simulink library "Lib_JMplatform_deVCU_Com"  (R2019b)
settings: Solver=ode45  StartTime=0.0  StopTime=10.0  RelTol=1e-3  EnableMultiTasking=on
settings Model: Creator=kmansour  LastModifiedBy=User
settings DataIOCC: LimitDataPoints=on  SaveFormat=Array  ReturnWorkspaceOutputs=off
settings OptimizationCC: LifeSpan=inf
settings DebuggingCC: AllowSymbolicDim=off  SFUnexpectedBacktrackingDiag=warning  SFNoUnconditionalDefaultTransitionDiag=warning  SFExecutionAtInitializationDiag=none  ArithmeticOperatorsInVariantConditions=warning
settings HardwareCC: ProdBitPerPointer=32  ProdBitPerSizeT=32  ProdBitPerPtrDiffT=32  ProdLargestAtomicFloat=None  ProdIntDivRoundTo=Undefined  ProdEndianess=Unspecified  ProdWordSize=32  ProdHWDeviceType=32-bit Generic
settings ModelReferenceCC: PropagateSignalLabelsOutOfModel=off
settings SFSimCC: SimUseLocalCustomCode=off  CustomCodeUndefinedFunction=UseInterfaceOnly
settings RTWCC: RTWUseLocalCustomCode=off
settings CodeAppCC: StateflowObjectComments=on
settings GRTTargetCC: TargetLangStandard=C89/C90 (ANSI)  GeneratePreprocessorConditionals=Disable all
settings ConfigComp: CovMetricSettings=dw  CovHtmlReporting=on  CovSaveCumulativeToWorkspaceVar=on  CovSaveSingleToWorkspaceVar=on  CovExternalEMLEnable=off

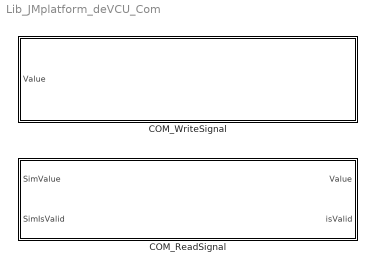
== system Lib_JMplatform_deVCU_Com ==
  COM_ReadSignal : Subsystem  TreatAsAtomicUnit=on  mask{PARAM_ID=APP_RX_CAN1TESTRX1}
      mask prompts: PARAM_ID "Choose Signal"
      mask TypeOptions PARAM_ID: APP_RX_CAN1TESTRX1 | APP_RX_CAN2TESTRX1 | APP_RX_CAN3TESTRX1
      mask Display:
      | image(imread('devcu_final.png'),'top-left');
      | color('black');
      | port_label('input', 1, 'SimValue');
      | port_label('input', 2, 'SimIsValid');
      | port_label('output', 1, 'Value');
      | port_label('output', 2, 'isValid');
      | 
      | strCell =get_param(gcb, 'MaskValues');
      | strCell = strtrim(strCell);
      | str = strCell{1};
      | str = strrep(str, '_', '\_');
      | disp(str, 'texmode', 'on');
  COM_WriteSignal : Subsystem  TreatAsAtomicUnit=on  mask{PARAM_ID=APP_TX_CAN1TESTTX1}
      mask prompts: PARAM_ID "Choose Signal"
      mask TypeOptions PARAM_ID: APP_TX_CAN1TESTTX1 | APP_TX_CAN2TESTTX2 | APP_TX_CAN3TEXTTX1
      mask Display:
      | image(imread('devcu_final.png'),'top-right');
      | color('black');
      | port_label('input', 1, 'Value');
      | 
      | strCell =get_param(gcb, 'MaskValues');
      | strCell = strtrim(strCell);
      | str = strCell{1};
      | str = strrep(str, '_', '\_');
      | disp(str, 'texmode', 'on');

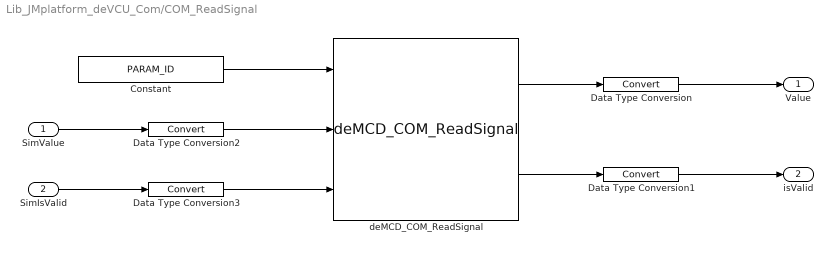
== system Lib_JMplatform_deVCU_Com/COM_ReadSignal ==
  SimValue : Inport
  SimIsValid : Inport  Port=2
  Constant : Constant  Value=PARAM_ID
  Data Type Conversion{,1..3} (4 alike) : DataTypeConversion
  deMCD_COM_ReadSignal : S-Function  FunctionName=deMCD_COM_ReadSignal  SFunctionDeploymentMode=off  EnableBusSupport=off
      mask Display:
      | image(imread('logo_deMCD_white_background.png'),'center');
      | color('black');
      | port_label('input', 1, 'ID');
      | port_label('input', 2, 'SimValue');
      | port_label('input', 3, 'SimIsValid');
      | port_label('output', 1, 'Value');
      | port_label('output', 2, 'isValid');
  Value : Outport
  isValid : Outport  Port=2
  wires:
  Constant/1 -> deMCD_COM_ReadSignal/1
  deMCD_COM_ReadSignal/1 -> Data Type Conversion/1
  deMCD_COM_ReadSignal/2 -> Data Type Conversion1/1
  Data Type Conversion/1 -> Value/1
  Data Type Conversion1/1 -> isValid/1
  SimValue/1 -> Data Type Conversion2/1
  Data Type Conversion2/1 -> deMCD_COM_ReadSignal/2
  Data Type Conversion3/1 -> deMCD_COM_ReadSignal/3
  SimIsValid/1 -> Data Type Conversion3/1

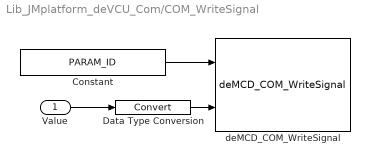
== system Lib_JMplatform_deVCU_Com/COM_WriteSignal ==
  Value : Inport
  Constant : Constant  Value=PARAM_ID
  Data Type Conversion : DataTypeConversion
  deMCD_COM_WriteSignal : S-Function  FunctionName=deMCD_COM_WriteSignal  SFunctionDeploymentMode=off  EnableBusSupport=off
      mask Display:
      | image(imread('logo_deMCD_white_background.png'),'center');
      | color('black');
      | port_label('input', 1, 'ID');
      | port_label('input', 2, 'Value');
  wires:
  Value/1 -> Data Type Conversion/1
  Constant/1 -> deMCD_COM_WriteSignal/1
  Data Type Conversion/1 -> deMCD_COM_WriteSignal/2
